simulink model "Stopwatch2"  (Simulink 5.0)
settings: Solver=FixedStepDiscrete  StartTime=0.0  StopTime=100000.0  RelTol=1e-3
libraries: simulink x2
settings Model: Creator=scaife  LastModifiedBy=scaife  ExtModeAutoUpdateStatusClock=off

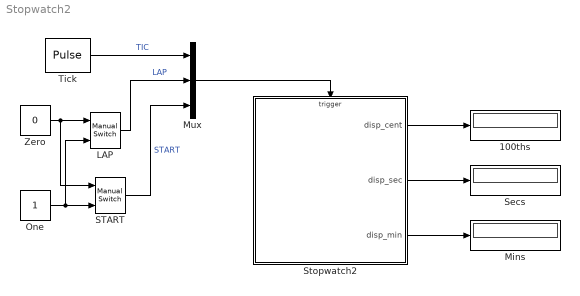
== system Stopwatch2 ==
  100ths : Display
  LAP : simulink/Signal Routing/Manual Switch  sw=1  action=0
  Mins : Display
  Mux : Mux  Inputs=3
  One : Constant
  START : simulink/Signal Routing/Manual Switch  sw=1  action=0
  Secs : Display
  Stopwatch2 : Stateflow chart
  Tick : DiscretePulseGenerator  SampleTime=0.01  VectorParams1D=off
  Zero : Constant  Value=0
  wires:
  Stopwatch2/1(disp_cent) -> 100ths/1
  Stopwatch2/2(disp_sec) -> Secs/1
  Stopwatch2/3(disp_min) -> Mins/1
  Tick/1 -> Mux/1  "TIC"
  Zero/1 -> LAP/1, START/1
  One/1 -> START/2, LAP/2
  LAP/1 -> Mux/2  "LAP"
  Mux/1 -> Stopwatch2/Trigger
  START/1 -> Mux/3  "START"

== stateflow chart Stopwatch2 ==
  state Stop
    state Lap_stop
    state Reset/
      on LAP:
      cent=0; sec=0; min=0;
      disp_cent=0; disp_sec=0;
      disp_min=0;
    (default) -> Reset
    Lap_stop -> Reset : LAP
  state Run
    state Lap
    state Running/
      du:
      disp_cent=cent;
      disp_sec=sec;
      disp_min=min;
    Running -> Lap : LAP
    Run -> (junction 9) : TIC{cent++;}
    (junction 9) -> (junction 10) : [cent==100]{cent=0; sec++;}
    (junction 9) -> (junction 11)
    (junction 10) -> (junction 11)
    (junction 10) -> (junction 11) : [sec==60]{sec=0; min++;}
    Lap -> Running : LAP
  Reset -> Running : START
  Lap -> Lap_stop : START
  (default) -> Stop
  Running -> Reset : START
  Lap_stop -> Lap : START
  data: runlap local int32 =1; cent local int32; sec local int32; min local int32; disp_cent output int32; disp_sec output int32; disp_min output int32
  events: TIC input EITHER_EDGE_EVENT; LAP input EITHER_EDGE_EVENT; START input EITHER_EDGE_EVENT
